simulink model "model_3dof"  (R2018a)
settings: Solver=FixedStepAuto  StartTime=0.0  StopTime=10  FixedStep=1/Fs  RelTol=1e-3
values from neighbouring files (symbols this model uses):
  C1 = 10    [symulacja.m]
  C2 = 1    [symulacja.m]
  C3 = 10    [symulacja.m]
  Fs = 10000    [symulacja.m]
  K1 = 200000    [symulacja.m]
  K2 = 4000000    [symulacja.m]
  K3 = 600000    [symulacja.m]
libraries: simulink x3
settings Model: Creator=P  LastModifiedBy=Ancymon

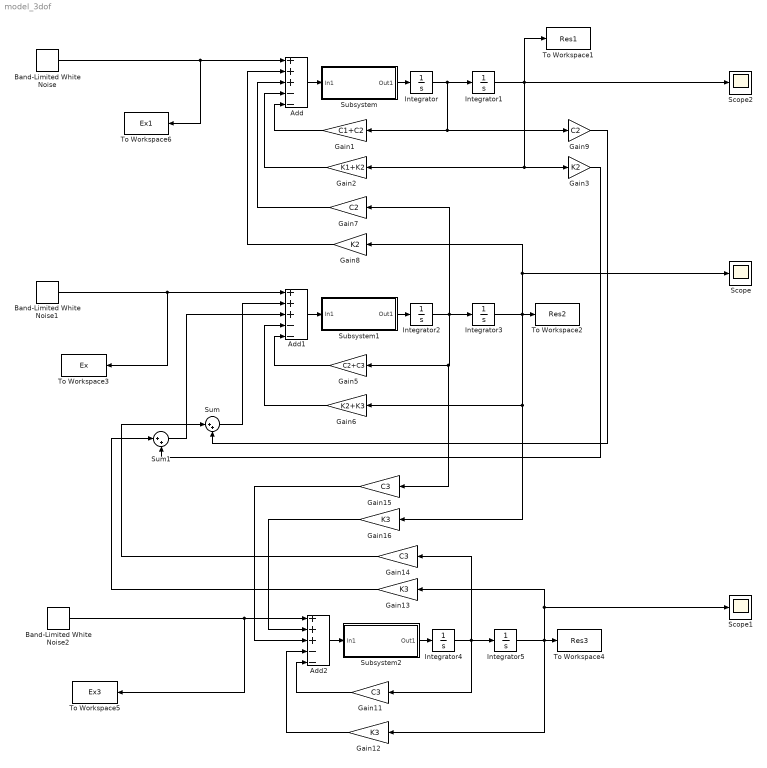
== system model_3dof ==
  Add : Sum  Inputs=+++--
  Add1 : Sum  Inputs=+++--
  Add2 : Sum  Inputs=+++--
  Band-Limited White Noise : simulink/Sources/Band-Limited White Noise  Cov=[0.1]  Ts=1/Fs  seed=[23341]
  Band-Limited White Noise1 : simulink/Sources/Band-Limited White Noise  Cov=[0.1]  Ts=1/Fs  seed=[23341]
  Band-Limited White Noise2 : simulink/Sources/Band-Limited White Noise  Cov=[0.1]  Ts=1/Fs  seed=[23341]
  Gain1 : Gain  Gain=C1+C2
  Gain11 : Gain  Gain=C3
  Gain12 : Gain  Gain=K3
  Gain13 : Gain  Gain=K3
  Gain14 : Gain  Gain=C3
  Gain15 : Gain  Gain=C3
  Gain16 : Gain  Gain=K3
  Gain2 : Gain  Gain=K1+K2
  Gain3 : Gain  Gain=K2
  Gain5 : Gain  Gain=C2+C3
  Gain6 : Gain  Gain=K2+K3
  Gain7 : Gain  Gain=C2
  Gain8 : Gain  Gain=K2
  Gain9 : Gain  Gain=C2
  Integrator{,1..5} (6 alike) : Integrator
  Scope : Scope
  Scope1 : Scope
  Scope2 : Scope
  Subsystem : Subsystem
  Subsystem1 : Subsystem
  Subsystem2 : Subsystem
  Sum : Sum  Inputs=|++
  Sum1 : Sum  Inputs=|++
  To Workspace1 : ToWorkspace  VariableName=Res1  SampleTime=-1
  To Workspace2 : ToWorkspace  VariableName=Res2  SampleTime=-1
  To Workspace3 : ToWorkspace  VariableName=Ex  SampleTime=-1
  To Workspace4 : ToWorkspace  VariableName=Res3  SampleTime=-1
  To Workspace5 : ToWorkspace  VariableName=Ex3  SampleTime=-1
  To Workspace6 : ToWorkspace  VariableName=Ex1  SampleTime=-1
  wires:
  Integrator/1 -> Gain9/1, Gain1/1, Integrator1/1
  Gain1/1 -> Add/5
  Gain2/1 -> Add/4
  Integrator1/1 -> Scope2/1, To Workspace1/1, Gain3/1, Gain2/1
  Integrator2/1 -> Gain7/1, Gain15/1, Gain5/1, Integrator3/1
  Integrator3/1 -> Gain8/1, Scope/1, Gain16/1, Gain6/1, To Workspace2/1
  Gain5/1 -> Add1/5
  Gain6/1 -> Add1/4
  Gain7/1 -> Add/3
  Gain8/1 -> Add/2
  Gain3/1 -> Sum1/2
  Gain9/1 -> Sum/2
  Band-Limited White Noise/1 -> To Workspace6/1, Add/1
  Band-Limited White Noise1/1 -> To Workspace3/1, Add1/1
  Band-Limited White Noise2/1 -> To Workspace5/1, Add2/1
  Integrator4/1 -> Gain14/1, Gain11/1, Integrator5/1
  Gain11/1 -> Add2/5
  Gain12/1 -> Add2/4
  Integrator5/1 -> Scope1/1, Gain13/1, Gain12/1, To Workspace4/1
  Gain14/1 -> Sum/1
  Gain13/1 -> Sum1/1
  Sum/1 -> Add1/2
  Sum1/1 -> Add1/3
  Gain15/1 -> Add2/3
  Gain16/1 -> Add2/2
  Subsystem/1(Out1) -> Integrator/1
  Add/1 -> Subsystem/1(In1)
  Add2/1 -> Subsystem2/1(In1)
  Subsystem2/1(Out1) -> Integrator4/1
  Add1/1 -> Subsystem1/1(In1)
  Subsystem1/1(Out1) -> Integrator2/1

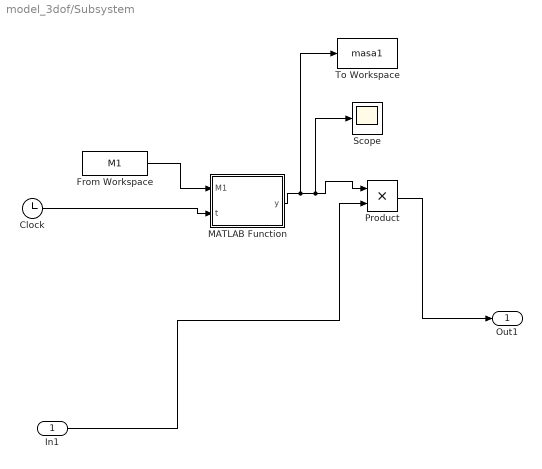
== system model_3dof/Subsystem ==
  In1 : Inport
  Clock : Clock
  From Workspace : FromWorkspace  VariableName=M1  SampleTime=0
  MATLAB Function : MATLAB Function  TreatAsAtomicUnit=on
  Product : Product
  Scope : Scope
  To Workspace : ToWorkspace  VariableName=masa1  SampleTime=-1
  Out1 : Outport
  wires:
  Clock/1 -> MATLAB Function/2(t)
  MATLAB Function/1(y) -> To Workspace/1, Product/1, Scope/1
  Product/1 -> Out1/1
  In1/1 -> Product/2
  From Workspace/1 -> MATLAB Function/1(M1)

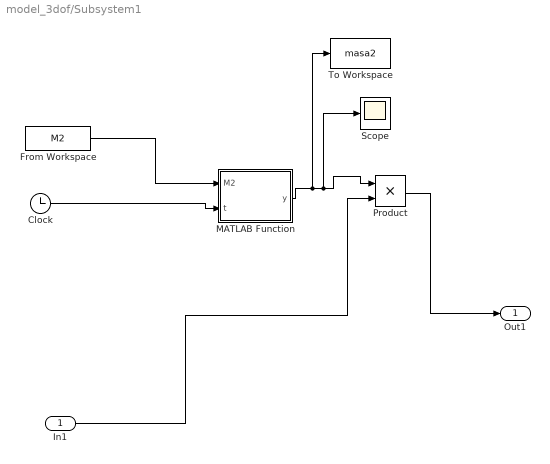
== system model_3dof/Subsystem1 ==
  In1 : Inport
  Clock : Clock
  From Workspace : FromWorkspace  VariableName=M2  SampleTime=0
  MATLAB Function : MATLAB Function  TreatAsAtomicUnit=on
  Product : Product
  Scope : Scope
  To Workspace : ToWorkspace  VariableName=masa2  SampleTime=-1
  Out1 : Outport
  wires:
  Clock/1 -> MATLAB Function/2(t)
  MATLAB Function/1(y) -> To Workspace/1, Product/1, Scope/1
  Product/1 -> Out1/1
  In1/1 -> Product/2
  From Workspace/1 -> MATLAB Function/1(M2)

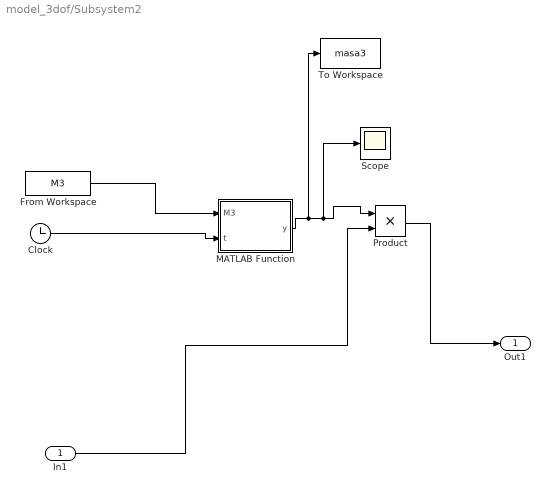
== system model_3dof/Subsystem2 ==
  In1 : Inport
  Clock : Clock
  From Workspace : FromWorkspace  VariableName=M3  SampleTime=0
  MATLAB Function : MATLAB Function  TreatAsAtomicUnit=on
  Product : Product
  Scope : Scope
  To Workspace : ToWorkspace  VariableName=masa3  SampleTime=-1
  Out1 : Outport
  wires:
  Clock/1 -> MATLAB Function/2(t)
  MATLAB Function/1(y) -> To Workspace/1, Product/1, Scope/1
  Product/1 -> Out1/1
  In1/1 -> Product/2
  From Workspace/1 -> MATLAB Function/1(M3)

== matlab function model_3dof/Subsystem/MATLAB Function ==
  data: M1 input; y output; t input
function y = fcn(M1,t)

y = 1/(M1+20*t);

== matlab function model_3dof/Subsystem1/MATLAB Function ==
  data: M2 input; y output; t input
function y = fcn(M2,t)

y = 1/abs(M2+80*t);

== matlab function model_3dof/Subsystem2/MATLAB Function ==
  data: M3 input; y output; t input
function y = fcn(M3,t)

y = 1/abs(M3-40*t);
